simulink library "CommercialVehicleLibrary2G"  (R2021a)
settings: Solver=VariableStepAuto  StartTime=0.0  StopTime=10.0  RelTol=1e-3
values from neighbouring files (symbols this model uses):
  brake_input = [0   tmax ... (first row only)    [init_vehicle.m]    (also in run_Circle.m = [0  tmax; run_Coastdown.m = [0  2  tmax; run_DoubleLaneChangeDriver.m = [0   2  tmax; run_MaxAcc.m = [0  2  tmax)
  pose_t0 = [0 0 0 0]    [init_vehicle.m]    (also in run_Circle.m; run_Coastdown.m; run_DoubleLaneChangeDriver.m; run_MaxAcc.m)
  rdfname = 'TNO_FlatRoad.rdf'    [run_Circle.m]    (also in run_Coastdown.m; run_DoubleLaneChangeDriver.m; run_MaxAcc.m; run_Rollover.m)
  rdfname_inner = 'TNO_FlatRoad.rdf'    [run_Circle.m]    (also in run_Coastdown.m; run_DoubleLaneChangeDriver.m; run_MaxAcc.m; run_Rollover.m)
  steer_input = [0  tmax ... (first row only)    [init_vehicle.m]    (also in run_Circle.m = [0  2   10     13       tmax; run_Coastdown.m = [0 tmax; run_DoubleLaneChangeDriver.m = [0 tmax; run_MaxAcc.m = [0 tmax)
  throttle_input = [0         tmax ... (first row only)    [init_vehicle.m]    (also in run_Circle.m; run_Coastdown.m = [0        10         10.0001 tmax; run_DoubleLaneChangeDriver.m = [0        tmax; run_MaxAcc.m = [0        tmax)
  Vx = 0    [init_vehicle.m]    (also in run_Circle.m = Vx_kmh/3.6; run_Coastdown.m = Vx_kmh/3.6; run_DoubleLaneChangeDriver.m = Vx_kmh/3.6; run_MaxAcc.m)
  Vx_input = [0  tmax ... (first row only)    [init_vehicle.m]    (also in run_Circle.m; run_Coastdown.m = [0 tmax; run_DoubleLaneChangeDriver.m = [0 tmax; run_MaxAcc.m = [0 tmax)
undefined symbols (not defined in the file or in its folder): Drive, Floor, Fzstat, Fzstat1, Fzstat3, l, l_load1, l_load2, lbar, mass_load1, mass_load2, psi_semitrailer, rho, rim_Ixx, rim_Iyy, rim_mass, Steer, steer_path, tpfname, X, x_torsion, xcg, xcg1, xcg2, xcg_front, xcg_rear, xdrive1, xload1, xload2, xpos1, xref, xrev1, Xt0, Y, Yt0, Z
libraries: sm_lib x291, $bdroot x157, nesl_utility x143, vrlib x1
(part 10 of 12)

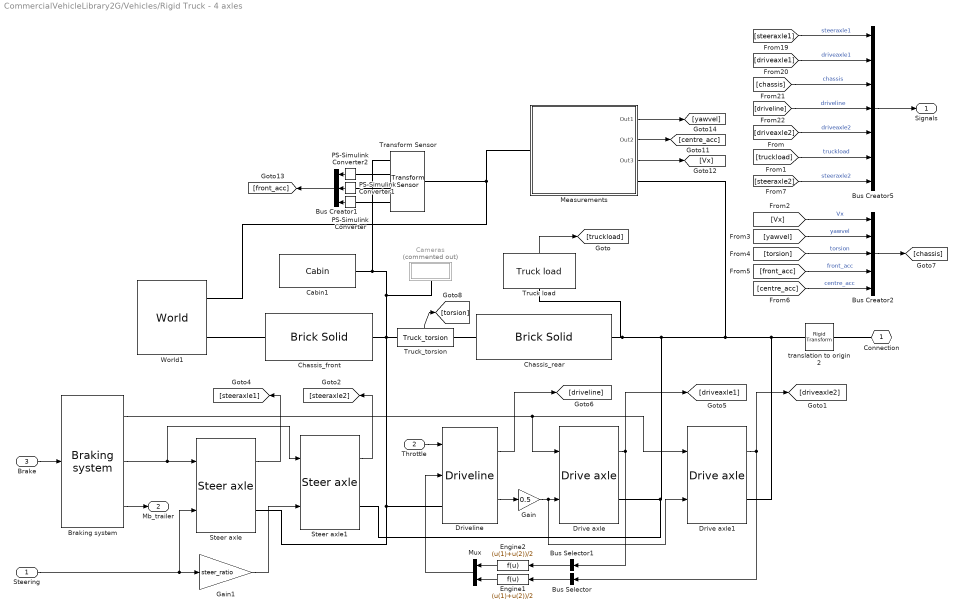
== system CommercialVehicleLibrary2G/Vehicles/Rigid Truck - 4 axles ==
  Steering : Inport
  Throttle : Inport  Port=2
  Brake : Inport  Port=3
  Braking system : $bdroot/Components/Braking system  SystemSampleTime=-1  VariantActivationTime=update diagram  Latency=0  AutoFrameSizeCalculation=off
  Bus Creator1 : BusCreator  Inputs=3
  Bus Creator2 : BusCreator  Inputs=5
  Bus Creator5 : BusCreator  Inputs=7
  Bus Selector : BusSelector  OutputSignals=Omega1,Omega2  OutputAsBus=on
  Bus Selector1 : BusSelector  OutputSignals=Omega1,Omega2  OutputAsBus=on
  Cabin1 : $bdroot/Assemblies/Cabin  xref=xref+1.10  zref=1.20
  Cameras : Subsystem  Commented=on
      settings: PortSchema="{\"entries\":[{\"content\":{\"sides\":[{\"content\":{\"connectorIds\":[]},\"type\":\"ConnectorPlacement.EquallySpacedRectSide\",\"uuid\":\"a276cb58-0a92-429b-8e88-be3307b37bb7\"},{\"content\":{\"connectorIds\":[],\"side\":\"RIGHT\"},\"type\":\"ConnectorPlacement.EquallySpacedRectSide\",\"uuid\":\"8a90bce0-2fe2-4c94-b803-8b8b0449a6a1\"},{\"content\":{\"connectorIds\":[],\"side\":\"TOP\"},\"type\":\"ConnectorPlacement.EquallySpacedRectSide\",\"uuid\":\"98d3107c-5bc7-4afe-b9f8-41acdc56c58c\"},{\"content\":{\"connectorIds\":[\"RConn1\"],\"side\":\"BOTTOM\"},\"type\":\"ConnectorPlacement.EquallySpacedRectSide\",\"uuid\":\"24ac9801-a810-4d3b-b9e2-6521fa5912b6\"}]},\"type\":\"ConnectorPlacement.EquallySpacedConnector\",\"uuid\":\"603d60ad-e553-44b7-87a5-94eb629e36a6\"}],\"packageUris\":[\"http://schema.mathworks.com/mf0/Connector/R2020b\"],\"version\":\"1.0\"}"
  Chassis_front : sm_lib/Body Elements/Brick Solid  GraphicAmbientColor=[0.15 0.15 0.15 1.0]  BasedOnType=Density  BrickDimensions=[l1 w1 h1]  BrickDimensionUnits=m  CenterOfMass=[0 0 0]  CenterOfMassUnits=m  GraphicDiffuseColor=[0.9 0.9 0.9]  Density=1000  DensityUnits=kg/m^3  DoExposeReferenceFrame=on  GraphicEmissiveColor=[0.0 0.0 0.0 1.0]  ExportEntireGeometry=off  SerializedFrames=<Frames><Frame><Id>Frame1</Id><Value><Name>F1</Name><Origin><Source>ReferenceFrame</Source><FeatureName></FeatureName></Origin><PrimaryAxis><DefinedDirection>+Z</DefinedDirection><Source>ReferenceFrame</Source><SourceDirection>+Z</SourceDirection><FeatureName></FeatureName></PrimaryAxis><SecondaryAxis><DefinedDirection>+X</DefinedDirection><Source>ReferenceFrame</Source><SourceDirection>+X</SourceDirection><FeatureName></FeatureName></SecondaryAxis></Value></Frame></Frames>  MarkerShape=Sphere  MarkerSize=10  GraphicType=FromGeometry  InertiaType=Custom  Mass=front_mass  MassUnits=kg  MomentsOfInertia=[front_Ixx front_Iyy front_Izz]  MomentsOfInertiaUnits=kg*m^2  GraphicOpacity=0.8  ProductsOfInertia=[0 0 0]  ProductsOfInertiaUnits=kg*m^2  GraphicShininess=75  GraphicSpecularColor=[0.5 0.5 0.5 1.0]  GraphicVisPropType=SimpleVisualProperties
  Chassis_rear : sm_lib/Body Elements/Brick Solid  GraphicAmbientColor=[0.15 0.15 0.15 1.0]  BasedOnType=Density  BrickDimensions=[l2 w2 h2]  BrickDimensionUnits=m  CenterOfMass=[0 0 0]  CenterOfMassUnits=m  GraphicDiffuseColor=[0.9 0.9 0.9]  Density=1000  DensityUnits=kg/m^3  DoExposeReferenceFrame=on  GraphicEmissiveColor=[0.0 0.0 0.0 1.0]  ExportEntireGeometry=off  SerializedFrames=<Frames><Frame><Id>Frame1</Id><Value><Name>F1</Name><Origin><Source>ReferenceFrame</Source><FeatureName></FeatureName></Origin><PrimaryAxis><DefinedDirection>+Z</DefinedDirection><Source>ReferenceFrame</Source><SourceDirection>+Z</SourceDirection><FeatureName></FeatureName></PrimaryAxis><SecondaryAxis><DefinedDirection>+X</DefinedDirection><Source>ReferenceFrame</Source><SourceDirection>+X</SourceDirection><FeatureName></FeatureName></SecondaryAxis></Value></Frame></Frames>  MarkerShape=Sphere  MarkerSize=10  GraphicType=FromGeometry  InertiaType=Custom  Mass=rear_mass  MassUnits=kg  MomentsOfInertia=[rear_Ixx rear_Iyy rear_Izz]  MomentsOfInertiaUnits=kg*m^2  GraphicOpacity=0.8  ProductsOfInertia=[0 0 0]  ProductsOfInertiaUnits=kg*m^2  GraphicShininess=75  GraphicSpecularColor=[0.5 0.5 0.5 1.0]  GraphicVisPropType=SimpleVisualProperties
  Drive axle : $bdroot/Assemblies/Drive axle  xpos=xdrive1  tpfname='truck1.tpf'  rdfname=rdfname  rdfname_inner=rdfname_inner  Vx=Vx  Fzstat=Fzstat3
  Drive axle1 : $bdroot/Assemblies/Drive axle  xpos=xdrive2  tpfname='truck1.tpf'  rdfname=rdfname  rdfname_inner=rdfname_inner  Vx=Vx  Fzstat=Fzstat4
  Driveline : $bdroot/Assemblies/Driveline  xref=xref-0.162  zref=0.58  param=DAF XEC + TC-Tronic (355 kW/2100 Nm)
  Engine1 : Fcn  Expr=(u(1)+u(2))/2
  Engine2 : Fcn  Expr=(u(1)+u(2))/2
  Gain : Gain  Gain=0.5
  Gain1 : Gain  Gain=steer_ratio
  Measurements : Subsystem
  Mux : Mux  Inputs=2
  PS-Simulink Converter : nesl_utility/PS-Simulink Converter  PhysicalDomain=network_engine_domain  SubClassName=ps_output  LeftPortType=input  RightPortType=output  PseudoPeriodic=off  Frequencies=[]  Unit=inherit  AffineConversion=off
  PS-Simulink Converter1 : nesl_utility/PS-Simulink Converter  PhysicalDomain=network_engine_domain  SubClassName=ps_output  LeftPortType=input  RightPortType=output  PseudoPeriodic=off  Frequencies=[]  Unit=inherit  AffineConversion=off
  PS-Simulink Converter2 : nesl_utility/PS-Simulink Converter  PhysicalDomain=network_engine_domain  SubClassName=ps_output  LeftPortType=input  RightPortType=output  PseudoPeriodic=off  Frequencies=[]  Unit=inherit  AffineConversion=off
  Steer axle : $bdroot/Assemblies/Steer axle  xpos=xref  tpfname='truck2b2.tpf'  rdfname=rdfname  Vx=Vx  Fzstat=Fzstat1
  Steer axle1 : $bdroot/Assemblies/Steer axle  xpos=xsteer2-xcg_rear  tpfname='truck2b2.tpf'  rdfname=rdfname  Vx=Vx  Fzstat=Fzstat2
  Transform Sensor : sm_lib/Frames and Transforms/Transform Sensor  MeasurementFrame=NonRotatingFollower  SenseAngle=off  SenseAxis=off  SenseAngle1=off  SenseAngle2=off  SenseAngle3=off  SenseQ=off  SenseR=off  SenseOmegaX=off  SenseOmegaY=off  SenseOmegaZ=off  SenseOmega1=off  SenseOmega2=off  SenseOmega3=off  SenseQDot=off  SenseRDot=off  SenseAlphaX=off  SenseAlphaY=off  SenseAlphaZ=off  SenseAlpha1=off  SenseAlpha2=off  SenseAlpha3=off  SenseQDDot=off  SenseRDDot=off  SenseX=off  SenseY=off  SenseZ=off  SenseRad=off  SenseAzim=off  SenseDist=off  SenseInc=off  SenseXDot=off  SenseYDot=off  SenseZDot=off  SenseRadDot=off  SenseAzimDot=off  SenseDistDot=off  SenseIncDot=off  SenseXDDot=on  SenseYDDot=on  SenseZDDot=on  SenseRadDDot=off  SenseAzimDDot=off  SenseDistDDot=off  SenseIncDDot=off
  Truck load : $bdroot/Assemblies/Truck load  xload=xload  zload=1.3  mass_load=mass_load  l_load=l_load  w=2.5  rho=rho
  Truck_torsion : $bdroot/Components/Truck_torsion  SystemSampleTime=-1  VariantActivationTime=update diagram  Latency=0  AutoFrameSizeCalculation=off
      settings: PortSchema="{\"entries\":[{\"content\":{\"sides\":[{\"content\":{\"connectorIds\":[\"LConn1\"]},\"type\":\"ConnectorPlacement.EquallySpacedRectSide\",\"uuid\":\"b43c74bd-af15-4ffb-863b-6a132848d787\"},{\"content\":{\"connectorIds\":[\"RConn1\"],\"side\":\"RIGHT\"},\"type\":\"ConnectorPlacement.EquallySpacedRectSide\",\"uuid\":\"8ef5ae9f-2f99-4b38-816f-c2fb0756fe1b\"},{\"content\":{\"connectorIds\":[\"Out1\"],\"side\":\"TOP\"},\"type\":\"ConnectorPlacement.EquallySpacedRectSide\",\"uuid\":\"649c363b-e78d-45fa-ac8c-bda3eda724e3\"}]},\"type\":\"ConnectorPlacement.EquallySpacedConnector\",\"uuid\":\"06fb9ebd-5177-4420-93bb-82569f181fb4\"}],\"packageUris\":[\"http://schema.mathworks.com/mf0/Connector/R2020b\"],\"version\":\"1.0\"}"
  World1 : $bdroot/Utilities/World  SystemSampleTime=-1  VariantActivationTime=update diagram  Latency=0  AutoFrameSizeCalculation=off
  translation to origin 2 : sm_lib/Frames and Transforms/Rigid Transform  TranslationMethod=Cartesian  TranslationStandardOffset=0  TranslationLengthUnit=m  TranslationStandardAxis=+Z  TranslationCartesianOffset=[-xcg_rear 0 -0.9]  TranslationROffset=0  TranslationROffsetUnits=m  TranslationZOffset=0  TranslationZOffsetUnits=m  TranslationThetaOffset=0  TranslationThetaOffsetUnits=deg  RotationMethod=None  RotationAngleUnits=deg  RotationStandardAxis=+Z  RotationAngle=0.0  RotationArbitraryAxis=[0 0 1]  FollAlignAxisA=+Z  BaseAlignAxisA=+X  FollAlignAxisB=+Y  BaseAlignAxisB=+Y  RotationSequenceAxes=FollowerAxes  RotationSequence=XYX  RotationSequenceAngles=[0 0 0]  RotationSequenceAnglesUnits=deg  RotationMatrix=[1 0 0; 0 1 0; 0 0 1]
  Connection : PMIOPort  Tag=PMCPort  Side=Right
  Signals : Outport
  Mb_trailer : Outport  Port=2
  wires:
  [yawvel] -> Bus Creator2/2  "yawvel"
  Bus Creator2/1 -> [chassis]
  [centre_acc] -> Bus Creator2/5  "centre_acc"
  [torsion] -> Bus Creator2/3  "torsion"
  [Vx] -> Bus Creator2/1  "Vx"
  [front_acc] -> Bus Creator2/4  "front_acc"
  Bus Creator1/1 -> [front_acc]
  PS-Simulink Converter2/1 -> Bus Creator1/1
  Truck_torsion/1 -> [torsion]
  PS-Simulink Converter/1 -> Bus Creator1/3
  Measurements/3(Out3) -> [Vx]
  Measurements/1(Out1) -> [yawvel]
  PS-Simulink Converter1/1 -> Bus Creator1/2
  Measurements/2(Out2) -> [centre_acc]
  Steer axle/1 -> [steeraxle1]
  Drive axle/1 -> [driveaxle1], Bus Selector1/1
  Braking system/3 -> Mb_trailer/1
  Brake/1 -> Braking system/1
  Throttle/1 -> Driveline/1
  Driveline/2 -> Gain/1
  Steering/1 -> Steer axle/2, Gain1/1
  Driveline/1 -> [driveline]
  [steeraxle1] -> Bus Creator5/1  "steeraxle1"
  [driveaxle1] -> Bus Creator5/2  "driveaxle1"
  [chassis] -> Bus Creator5/3  "chassis"
  [driveline] -> Bus Creator5/4  "driveline"
  Bus Creator5/1 -> Signals/1
  Braking system/1 -> Drive axle1/1, Drive axle/1
  Braking system/2 -> Steer axle1/1, Steer axle/1
  Drive axle1/1 -> [driveaxle2], Bus Selector/1
  [driveaxle2] -> Bus Creator5/5  "driveaxle2"
  Gain/1 -> Drive axle1/2, Drive axle/2
  Truck load/1 -> [truckload]
  [truckload] -> Bus Creator5/6  "truckload"
  Engine2/1 -> Mux/1
  Engine1/1 -> Mux/2
  Mux/1 -> Driveline/2
  Bus Selector1/1 -> Engine2/1
  Bus Selector/1 -> Engine1/1
  Gain1/1 -> Steer axle1/2
  Steer axle1/1 -> [steeraxle2]
  [steeraxle2] -> Bus Creator5/7  "steeraxle2"
  connections:
  Connection/RConn1 -- translation to origin 2/RConn1
  World1/RConn2 -- Chassis_front/RConn1
  Chassis_rear/RConn1 -- Truck_torsion/RConn1
  Transform Sensor/RConn2 -- PS-Simulink Converter2/LConn1
  PS-Simulink Converter/LConn1 -- Transform Sensor/RConn4
  PS-Simulink Converter1/LConn1 -- Transform Sensor/RConn3
  Measurements/LConn1 -- World1/RConn1 -- Transform Sensor/LConn1
  Cabin1/RConn1 -- Transform Sensor/RConn1 -- Cameras/RConn1 -- Steer axle/RConn1 -- Driveline/LConn1 -- Chassis_front/LConn1 -- Truck_torsion/LConn1
  Measurements/RConn1 -- Truck load/LConn1 -- Chassis_rear/LConn1 -- Steer axle1/RConn1 -- Drive axle/RConn1 -- Drive axle1/RConn1 -- translation to origin 2/LConn1

== system CommercialVehicleLibrary2G/Vehicles/Tractor ==
  Steering : Inport
  Throttle : Inport  Port=2
  Brake : Inport  Port=3
  Braking system : $bdroot/Components/Braking system  SystemSampleTime=-1  VariantActivationTime=update diagram  Latency=0  AutoFrameSizeCalculation=off
  Bus Creator1 : BusCreator  Inputs=3
  Bus Creator2 : BusCreator  Inputs=5
  Bus Creator5 : BusCreator  Inputs=4
  Bus Selector : BusSelector  OutputSignals=Omega1,Omega2  OutputAsBus=on
  Cabin : $bdroot/Assemblies/Cabin  xref=xref+1.10  zref=1.20
  Cameras : Subsystem  Commented=on
  Chassis_front : sm_lib/Body Elements/Brick Solid  GraphicAmbientColor=[0.15 0.15 0.15 1.0]  BasedOnType=Density  BrickDimensions=[l1 w1 h1]  BrickDimensionUnits=m  CenterOfMass=[0 0 0]  CenterOfMassUnits=m  GraphicDiffuseColor=[0.4 0.4 0.4]  Density=1000  DensityUnits=kg/m^3  DoExposeReferenceFrame=on  GraphicEmissiveColor=[0.0 0.0 0.0 1.0]  ExportEntireGeometry=off  SerializedFrames=<Frames><Frame><Id>Frame1</Id><Value><Name>F1</Name><Origin><Source>ReferenceFrame</Source><FeatureName></FeatureName></Origin><PrimaryAxis><DefinedDirection>+Z</DefinedDirection><Source>ReferenceFrame</Source><SourceDirection>+Z</SourceDirection><FeatureName></FeatureName></PrimaryAxis><SecondaryAxis><DefinedDirection>+X</DefinedDirection><Source>ReferenceFrame</Source><SourceDirection>+X</SourceDirection><FeatureName></FeatureName></SecondaryAxis></Value></Frame></Frames>  MarkerShape=Sphere  MarkerSize=10  GraphicType=FromGeometry  InertiaType=Custom  Mass=front_mass  MassUnits=kg  MomentsOfInertia=[front_Ixx front_Iyy front_Izz]  MomentsOfInertiaUnits=kg*m^2  GraphicOpacity=1  ProductsOfInertia=[0 0 0]  ProductsOfInertiaUnits=kg*m^2  GraphicShininess=75  GraphicSpecularColor=[0.5 0.5 0.5 1.0]  GraphicVisPropType=SimpleVisualProperties
  Chassis_rear : sm_lib/Body Elements/Brick Solid  GraphicAmbientColor=[0.15 0.15 0.15 1.0]  BasedOnType=Density  BrickDimensions=[l2 w2 h2]  BrickDimensionUnits=m  CenterOfMass=[0 0 0]  CenterOfMassUnits=m  GraphicDiffuseColor=[0.9 0.9 0.9]  Density=1000  DensityUnits=kg/m^3  DoExposeReferenceFrame=on  GraphicEmissiveColor=[0.0 0.0 0.0 1.0]  ExportEntireGeometry=off  SerializedFrames=<Frames><Frame><Id>Frame1</Id><Value><Name>F1</Name><Origin><Source>ReferenceFrame</Source><FeatureName></FeatureName></Origin><PrimaryAxis><DefinedDirection>+Z</DefinedDirection><Source>ReferenceFrame</Source><SourceDirection>+Z</SourceDirection><FeatureName></FeatureName></PrimaryAxis><SecondaryAxis><DefinedDirection>+X</DefinedDirection><Source>ReferenceFrame</Source><SourceDirection>+X</SourceDirection><FeatureName></FeatureName></SecondaryAxis></Value></Frame></Frames>  MarkerShape=Sphere  MarkerSize=10  GraphicType=FromGeometry  InertiaType=Custom  Mass=rear_mass  MassUnits=kg  MomentsOfInertia=[rear_Ixx rear_Iyy rear_Izz]  MomentsOfInertiaUnits=kg*m^2  GraphicOpacity=0.8  ProductsOfInertia=[0 0 0]  ProductsOfInertiaUnits=kg*m^2  GraphicShininess=75  GraphicSpecularColor=[0.5 0.5 0.5 1.0]  GraphicVisPropType=SimpleVisualProperties
  Drive axle : $bdroot/Assemblies/Drive axle  xpos=xref+xrear  tpfname='truck1.tpf'  rdfname=rdfname  rdfname_inner=rdfname_inner  Vx=Vx  Fzstat=Fzstat2
  Driveline : $bdroot/Assemblies/Driveline  xref=xref-0.162  zref=0.58  param=DAF XEC + TC-Tronic (355 kW/2100 Nm)
  Measurements : Subsystem
  PS-Simulink Converter : nesl_utility/PS-Simulink Converter  PhysicalDomain=network_engine_domain  SubClassName=ps_output  LeftPortType=input  RightPortType=output  PseudoPeriodic=off  Frequencies=[]  Unit=inherit  AffineConversion=off
  PS-Simulink Converter1 : nesl_utility/PS-Simulink Converter  PhysicalDomain=network_engine_domain  SubClassName=ps_output  LeftPortType=input  RightPortType=output  PseudoPeriodic=off  Frequencies=[]  Unit=inherit  AffineConversion=off
  PS-Simulink Converter2 : nesl_utility/PS-Simulink Converter  PhysicalDomain=network_engine_domain  SubClassName=ps_output  LeftPortType=input  RightPortType=output  PseudoPeriodic=off  Frequencies=[]  Unit=inherit  AffineConversion=off
  Steer axle : $bdroot/Assemblies/Steer axle  xpos=xref  tpfname='truck2b2.tpf'  rdfname=rdfname  Vx=Vx  Fzstat=Fzstat1
  Tractor_torsion : $bdroot/Components/Tractor_torsion  SystemSampleTime=-1  VariantActivationTime=update diagram  Latency=0  AutoFrameSizeCalculation=off
      settings: PortSchema="{\"entries\":[{\"content\":{\"sides\":[{\"content\":{\"connectorIds\":[\"LConn1\"]},\"type\":\"ConnectorPlacement.EquallySpacedRectSide\",\"uuid\":\"b43c74bd-af15-4ffb-863b-6a132848d787\"},{\"content\":{\"connectorIds\":[\"RConn1\"],\"side\":\"RIGHT\"},\"type\":\"ConnectorPlacement.EquallySpacedRectSide\",\"uuid\":\"8ef5ae9f-2f99-4b38-816f-c2fb0756fe1b\"},{\"content\":{\"connectorIds\":[\"Out1\"],\"side\":\"TOP\"},\"type\":\"ConnectorPlacement.EquallySpacedRectSide\",\"uuid\":\"649c363b-e78d-45fa-ac8c-bda3eda724e3\"}]},\"type\":\"ConnectorPlacement.EquallySpacedConnector\",\"uuid\":\"06fb9ebd-5177-4420-93bb-82569f181fb4\"}],\"packageUris\":[\"http://schema.mathworks.com/mf0/Connector/R2020b\"],\"version\":\"1.0\"}"
  Transform Sensor : sm_lib/Frames and Transforms/Transform Sensor  MeasurementFrame=NonRotatingFollower  SenseAngle=off  SenseAxis=off  SenseAngle1=off  SenseAngle2=off  SenseAngle3=off  SenseQ=off  SenseR=off  SenseOmegaX=off  SenseOmegaY=off  SenseOmegaZ=off  SenseOmega1=off  SenseOmega2=off  SenseOmega3=off  SenseQDot=off  SenseRDot=off  SenseAlphaX=off  SenseAlphaY=off  SenseAlphaZ=off  SenseAlpha1=off  SenseAlpha2=off  SenseAlpha3=off  SenseQDDot=off  SenseRDDot=off  SenseX=off  SenseY=off  SenseZ=off  SenseRad=off  SenseAzim=off  SenseDist=off  SenseInc=off  SenseXDot=off  SenseYDot=off  SenseZDot=off  SenseRadDot=off  SenseAzimDot=off  SenseDistDot=off  SenseIncDot=off  SenseXDDot=on  SenseYDDot=on  SenseZDDot=on  SenseRadDDot=off  SenseAzimDDot=off  SenseDistDDot=off  SenseIncDDot=off
  World : $bdroot/Utilities/World  SystemSampleTime=-1  VariantActivationTime=update diagram  Latency=0  AutoFrameSizeCalculation=off
  translation to origin : sm_lib/Frames and Transforms/Rigid Transform  TranslationMethod=Cartesian  TranslationStandardOffset=0  TranslationLengthUnit=m  TranslationStandardAxis=+Z  TranslationCartesianOffset=[-xcg_rear 0 -0.9]  TranslationROffset=0  TranslationROffsetUnits=m  TranslationZOffset=0  TranslationZOffsetUnits=m  TranslationThetaOffset=0  TranslationThetaOffsetUnits=deg  RotationMethod=None  RotationAngleUnits=deg  RotationStandardAxis=+Z  RotationAngle=0.0  RotationArbitraryAxis=[0 0 1]  FollAlignAxisA=+Z  BaseAlignAxisA=+X  FollAlignAxisB=+Y  BaseAlignAxisB=+Y  RotationSequenceAxes=FollowerAxes  RotationSequence=XYX  RotationSequenceAngles=[0 0 0]  RotationSequenceAnglesUnits=deg  RotationMatrix=[1 0 0; 0 1 0; 0 0 1]
  5th Wheel : PMIOPort  Tag=PMCPort  Side=Right
  Signals : Outport
  Mb_trailer : Outport  Port=2
  wires:
  Braking system/2 -> Steer axle/1
  Braking system/1 -> Drive axle/1
  Bus Creator5/1 -> Signals/1
  [driveline] -> Bus Creator5/4  "driveline"
  [chassis] -> Bus Creator5/3  "chassis"
  [driveaxle] -> Bus Creator5/2  "driveaxle"
  [steeraxle] -> Bus Creator5/1  "steeraxle"
  Driveline/1 -> [driveline]
  Steering/1 -> Steer axle/2
  Driveline/2 -> Drive axle/2
  Bus Selector/1 -> Driveline/2
  Throttle/1 -> Driveline/1
  Brake/1 -> Braking system/1
  Braking system/3 -> Mb_trailer/1
  Drive axle/1 -> Bus Selector/1, [driveaxle]
  Steer axle/1 -> [steeraxle]
  Measurements/2(Out2) -> [centre_acc]
  PS-Simulink Converter1/1 -> Bus Creator1/2
  Measurements/1(Out1) -> [yawvel]
  Measurements/3(Out3) -> [Vx]
  PS-Simulink Converter/1 -> Bus Creator1/3
  Tractor_torsion/1 -> [torsion]
  PS-Simulink Converter2/1 -> Bus Creator1/1
  Bus Creator1/1 -> [front_acc]
  [front_acc] -> Bus Creator2/4  "front_acc"
  [Vx] -> Bus Creator2/1  "Vx"
  [torsion] -> Bus Creator2/3  "torsion"
  [centre_acc] -> Bus Creator2/5  "centre_acc"
  Bus Creator2/1 -> [chassis]
  [yawvel] -> Bus Creator2/2  "yawvel"
  connections:
  Cabin/RConn1 -- Cameras/LConn1 -- Transform Sensor/RConn1 -- Chassis_front/LConn1 -- Tractor_torsion/LConn1 -- Driveline/LConn1 -- Steer axle/RConn1
  Transform Sensor/LConn1 -- World/RConn1 -- Measurements/LConn1
  translation to origin/LConn1 -- Drive axle/RConn1 -- Chassis_rear/LConn1 -- Measurements/RConn1
  PS-Simulink Converter1/LConn1 -- Transform Sensor/RConn3
  PS-Simulink Converter/LConn1 -- Transform Sensor/RConn4
  Transform Sensor/RConn2 -- PS-Simulink Converter2/LConn1
  Chassis_rear/RConn1 -- Tractor_torsion/RConn1
  World/RConn2 -- Chassis_front/RConn1
  5th Wheel/RConn1 -- translation to origin/RConn1

== system CommercialVehicleLibrary2G/Assemblies/Cabin/Subsystem ==
  External Force and Torque : sm_lib/Forces and Torques/External Force and Torque  ForceResolutionFrame=AttachedFrame  EnableForceX=on  EnableForceY=off  EnableForceZ=off  EnableForce=off  TorqueResolutionFrame=AttachedFrame  EnableTorqueX=off  EnableTorqueY=off  EnableTorqueZ=off  EnableTorque=off
  Fcn : Fcn  Expr=-0.5*1.23*0.6*10.5*u(1)*abs(u(1))
  File Solid : sm_lib/Body Elements/File Solid  ExtGeomFileName=E:\Thesis\Original TST Model\Cabin.stl  UnitType=Custom  ExtGeomFileUnits=mm  StepReaderType=HEX  ExportConvexHullGeometry=off  InertiaType=Custom  Mass=1e-09  MassUnits=kg  CenterOfMass=[0 0 0]  CenterOfMassUnits=m  MomentsOfInertia=[1 1 1]  MomentsOfInertiaUnits=kg*m^2  ProductsOfInertia=[0 0 0]  ProductsOfInertiaUnits=kg*m^2  BasedOnType=DensityFromFile  Density=1000  DensityUnits=kg/m^3  DoExposeReferenceFrame=on  SerializedFrames=<Frames/>  GraphicType=FromGeometry  MarkerShape=Sphere  MarkerSize=10  GraphicVisPropType=SimpleVisualProperties  GraphicDiffuseColor=[0.4 0.4 0.4]  GraphicSpecularColor=[0.5 0.5 0.5 1.0]  GraphicAmbientColor=[0.15 0.15 0.15 1.0]  GraphicEmissiveColor=[0.0 0.0 0.0 1.0]  GraphicShininess=75  GraphicOpacity=1.0
  PS-Simulink Converter : nesl_utility/PS-Simulink Converter  PhysicalDomain=network_engine_domain  SubClassName=ps_output  LeftPortType=input  RightPortType=output  PseudoPeriodic=off  Frequencies=[]  Unit=inherit  AffineConversion=off
  Rigid Transform : sm_lib/Frames and Transforms/Rigid Transform  TranslationMethod=None  TranslationStandardOffset=0  TranslationLengthUnit=m  TranslationStandardAxis=+Z  TranslationCartesianOffset=[0 0 0]  TranslationROffset=0  TranslationROffsetUnits=m  TranslationZOffset=0  TranslationZOffsetUnits=m  TranslationThetaOffset=0  TranslationThetaOffsetUnits=deg  RotationMethod=StandardAxis  RotationAngleUnits=deg  RotationStandardAxis=+X  RotationAngle=90  RotationArbitraryAxis=[0 0 1]  FollAlignAxisA=+X  BaseAlignAxisA=+Y  FollAlignAxisB=+Y  BaseAlignAxisB=+Z  RotationSequenceAxes=FollowerAxes  RotationSequence=XYX  RotationSequenceAngles=[0 0 0]  RotationSequenceAnglesUnits=deg  RotationMatrix=[1 0 0; 0 1 0; 0 0 1]
  Rigid Transform3 : sm_lib/Frames and Transforms/Rigid Transform  TranslationMethod=None  TranslationStandardOffset=0  TranslationLengthUnit=m  TranslationStandardAxis=+Z  TranslationCartesianOffset=[0 0 0]  TranslationROffset=0  TranslationROffsetUnits=m  TranslationZOffset=0  TranslationZOffsetUnits=m  TranslationThetaOffset=0  TranslationThetaOffsetUnits=deg  RotationMethod=StandardAxis  RotationAngleUnits=deg  RotationStandardAxis=+Y  RotationAngle=90  RotationArbitraryAxis=[0 0 1]  FollAlignAxisA=+X  BaseAlignAxisA=+Y  FollAlignAxisB=+Y  BaseAlignAxisB=+Z  RotationSequenceAxes=FollowerAxes  RotationSequence=XYX  RotationSequenceAngles=[0 0 0]  RotationSequenceAnglesUnits=deg  RotationMatrix=[1 0 0; 0 1 0; 0 0 1]
  Rigid Transform4 : sm_lib/Frames and Transforms/Rigid Transform  TranslationMethod=Cartesian  TranslationStandardOffset=0  TranslationLengthUnit=m  TranslationStandardAxis=+Z  TranslationCartesianOffset=[0.15 -2.55 -1.75]  TranslationROffset=0  TranslationROffsetUnits=m  TranslationZOffset=0  TranslationZOffsetUnits=m  TranslationThetaOffset=0  TranslationThetaOffsetUnits=deg  RotationMethod=None  RotationAngleUnits=deg  RotationStandardAxis=+Y  RotationAngle=90  RotationArbitraryAxis=[0 0 1]  FollAlignAxisA=+X  BaseAlignAxisA=+Y  FollAlignAxisB=+Y  BaseAlignAxisB=+Z  RotationSequenceAxes=FollowerAxes  RotationSequence=XYX  RotationSequenceAngles=[0 0 0]  RotationSequenceAnglesUnits=deg  RotationMatrix=[1 0 0; 0 1 0; 0 0 1]
  Simulink-PS Converter : nesl_utility/Simulink-PS Converter  PhysicalDomain=network_engine_domain  SubClassName=ps_input  LeftPortType=input  RightPortType=output  PseudoPeriodic=off  Frequencies=[]  NoiseDistribution=none  NoiseParameters=[]  Unit=1  AffineConversion=off  FilteringAndDerivatives=provide  SimscapeFilterOrder=1  InputFilterTimeConstant=0.001  UdotUserProvided=0
  Transform Sensor : sm_lib/Frames and Transforms/Transform Sensor  MeasurementFrame=NonRotatingFollower  SenseAngle=off  SenseAxis=off  SenseAngle1=off  SenseAngle2=off  SenseAngle3=off  SenseQ=off  SenseR=off  SenseOmegaX=off  SenseOmegaY=off  SenseOmegaZ=off  SenseOmega1=off  SenseOmega2=off  SenseOmega3=off  SenseQDot=off  SenseRDot=off  SenseAlphaX=off  SenseAlphaY=off  SenseAlphaZ=off  SenseAlpha1=off  SenseAlpha2=off  SenseAlpha3=off  SenseQDDot=off  SenseRDDot=off  SenseX=off  SenseY=off  SenseZ=off  SenseRad=off  SenseAzim=off  SenseDist=off  SenseInc=off  SenseXDot=on  SenseYDot=off  SenseZDot=off  SenseRadDot=off  SenseAzimDot=off  SenseDistDot=off  SenseIncDot=off  SenseXDDot=off  SenseYDDot=off  SenseZDDot=off  SenseRadDDot=off  SenseAzimDDot=off  SenseDistDDot=off  SenseIncDDot=off
  World Frame : sm_lib/Frames and Transforms/World Frame
  Conn1 : PMIOPort  Side=Left
  wires:
  PS-Simulink Converter/1 -> Fcn/1
  Fcn/1 -> Simulink-PS Converter/1
  connections:
  Rigid Transform3/RConn1 -- Rigid Transform4/LConn1
  External Force and Torque/RConn1 -- File Solid/RConn1 -- Rigid Transform4/RConn1
  Transform Sensor/LConn1 -- World Frame/RConn1
  Simulink-PS Converter/RConn1 -- External Force and Torque/LConn1
  Transform Sensor/RConn1 -- Rigid Transform/LConn1 -- Conn1/RConn1
  PS-Simulink Converter/LConn1 -- Transform Sensor/RConn2
  Rigid Transform/RConn1 -- Rigid Transform3/LConn1

== system CommercialVehicleLibrary2G/Assemblies/Drive axle/Wheel 1 L ==
  MF Tyre L : $bdroot/Components/MF Tyre L  Tag=SimMechanics Wheel + tyre  idtyre=1  inertia=[rim_mass rim_Ixx rim_Iyy]  tpfname=tpfname  rdfname=rdfname  side_mode=(1xxx) left  cnt_mode=(x1xx) smooth road  dyn_mode=(xx1x) relaxation behaviour  mf_mode=(xxx4) combined  use_mode=1e8  disp_debug=off
  Non-moving road : $bdroot/Utilities/Non-moving road  Tag=Non-moving road  dummy=off
  Scaling factors : $bdroot/Utilities/Scaling factors  Tag=Scaling factors  LMUX=1  LKX=1  LMUY=1  LKY=1  LKYC=1  LTR=1  LKZC=1
  "Terminator " : Terminator
  B : PMIOPort  Side=Left
  Out1 : Outport
  wires:
  Non-moving road/1 -> MF Tyre L/1
  Scaling factors/1 -> MF Tyre L/2
  MF Tyre L/1 -> Out1/1
  MF Tyre L/2 -> "Terminator "/1
  connections:
  MF Tyre L/LConn1 -- B/RConn1

== system CommercialVehicleLibrary2G/Assemblies/Drive axle/Wheel 2 L ==
  2nd Wheel offset : sm_lib/Frames and Transforms/Rigid Transform  TranslationMethod=StandardAxis  TranslationStandardOffset=-ywhl  TranslationLengthUnit=m  TranslationStandardAxis=+Z  TranslationCartesianOffset=[0 0 0]  TranslationROffset=0  TranslationROffsetUnits=m  TranslationZOffset=0  TranslationZOffsetUnits=m  TranslationThetaOffset=0  TranslationThetaOffsetUnits=deg  RotationMethod=None  RotationAngleUnits=deg  RotationStandardAxis=+Z  RotationAngle=0.0  RotationArbitraryAxis=[0 0 1]  FollAlignAxisA=+X  BaseAlignAxisA=+Y  FollAlignAxisB=+Y  BaseAlignAxisB=+Z  RotationSequenceAxes=FollowerAxes  RotationSequence=XYX  RotationSequenceAngles=[0 0 0]  RotationSequenceAnglesUnits=deg  RotationMatrix=[1 0 0; 0 1 0; 0 0 1]
  MF Tyre L : $bdroot/Components/MF Tyre L  Tag=SimMechanics Wheel + tyre  idtyre=1  inertia=[rim_mass rim_Ixx rim_Iyy]  tpfname=tpfname  rdfname=rdfname  side_mode=(1xxx) left  cnt_mode=(x1xx) smooth road  dyn_mode=(xx1x) relaxation behaviour  mf_mode=(xxx4) combined  use_mode=1e8  disp_debug=off
  Non-moving road : $bdroot/Utilities/Non-moving road  Tag=Non-moving road  dummy=off
  Scaling factors : $bdroot/Utilities/Scaling factors  Tag=Scaling factors  LMUX=1  LKX=1  LMUY=1  LKY=1  LKYC=1  LTR=1  LKZC=1
  "Terminator " : Terminator
  B : PMIOPort  Side=Left
  Out1 : Outport
  wires:
  MF Tyre L/2 -> "Terminator "/1
  MF Tyre L/1 -> Out1/1
  Scaling factors/1 -> MF Tyre L/2
  Non-moving road/1 -> MF Tyre L/1
  connections:
  MF Tyre L/LConn1 -- 2nd Wheel offset/RConn1
  2nd Wheel offset/LConn1 -- B/RConn1

== system CommercialVehicleLibrary2G/Assemblies/Drive axle/Wheel1 R ==
  MF Tyre R : $bdroot/Components/MF Tyre R  Tag=SimMechanics Wheel + tyre  idtyre=2  inertia=[rim_mass rim_Ixx rim_Iyy]  tpfname=tpfname  rdfname=rdfname  side_mode=(2xxx) right  cnt_mode=(x1xx) smooth road  dyn_mode=(xx1x) relaxation behaviour  mf_mode=(xxx4) combined  use_mode=1e8  disp_debug=off
  Non-moving road : $bdroot/Utilities/Non-moving road  Tag=Non-moving road  dummy=off
  Scaling factors : $bdroot/Utilities/Scaling factors  Tag=Scaling factors  LMUX=1  LKX=1  LMUY=1  LKY=1  LKYC=1  LTR=1  LKZC=1
  Terminator 3 : Terminator
  B : PMIOPort  Side=Left
  Out1 : Outport
  wires:
  MF Tyre R/2 -> Terminator 3/1
  MF Tyre R/1 -> Out1/1
  Non-moving road/1 -> MF Tyre R/1
  Scaling factors/1 -> MF Tyre R/2
  connections:
  B/RConn1 -- MF Tyre R/LConn1

== system CommercialVehicleLibrary2G/Assemblies/Drive axle/Wheel2 R ==
  2nd Wheel offset : sm_lib/Frames and Transforms/Rigid Transform  TranslationMethod=StandardAxis  TranslationStandardOffset=ywhl  TranslationLengthUnit=m  TranslationStandardAxis=+Z  TranslationCartesianOffset=[0 0 0]  TranslationROffset=0  TranslationROffsetUnits=m  TranslationZOffset=0  TranslationZOffsetUnits=m  TranslationThetaOffset=0  TranslationThetaOffsetUnits=deg  RotationMethod=None  RotationAngleUnits=deg  RotationStandardAxis=+Z  RotationAngle=0.0  RotationArbitraryAxis=[0 0 1]  FollAlignAxisA=+X  BaseAlignAxisA=+Y  FollAlignAxisB=+Y  BaseAlignAxisB=+Z  RotationSequenceAxes=FollowerAxes  RotationSequence=XYX  RotationSequenceAngles=[0 0 0]  RotationSequenceAnglesUnits=deg  RotationMatrix=[1 0 0; 0 1 0; 0 0 1]
  MF Tyre R : $bdroot/Components/MF Tyre R  Tag=SimMechanics Wheel + tyre  idtyre=2  inertia=[rim_mass rim_Ixx rim_Iyy]  tpfname=tpfname  rdfname=rdfname  side_mode=(2xxx) right  cnt_mode=(x1xx) smooth road  dyn_mode=(xx1x) relaxation behaviour  mf_mode=(xxx4) combined  use_mode=1e8  disp_debug=off
  Non-moving road : $bdroot/Utilities/Non-moving road  Tag=Non-moving road  dummy=off
  Scaling factors : $bdroot/Utilities/Scaling factors  Tag=Scaling factors  LMUX=1  LKX=1  LMUY=1  LKY=1  LKYC=1  LTR=1  LKZC=1
  "Terminator " : Terminator
  B : PMIOPort  Side=Left
  Out1 : Outport
  wires:
  MF Tyre R/1 -> Out1/1
  MF Tyre R/2 -> "Terminator "/1
  Non-moving road/1 -> MF Tyre R/1
  Scaling factors/1 -> MF Tyre R/2
  connections:
  2nd Wheel offset/LConn1 -- B/RConn1
  2nd Wheel offset/RConn1 -- MF Tyre R/LConn1

== system CommercialVehicleLibrary2G/Assemblies/Driveline/engine and differential ==
  throttle : Inport
  omega_wheels : Inport  Port=2
  Bus Creator : BusCreator  Inputs=2
  Demux : Demux  Outputs=2
  Engine : Fcn  Expr=eng_power/(abs(u)+1e-10)
  Mux : Mux  Inputs=2
  Product2 : Product  Inputs=3  InputSameDT=on  SaturateOnIntegerOverflow=on  OutDataTypeStr=Inherit: Same as first input
  Saturation : Saturate  UpperLimit=max_engine_torque*first_gear_ratio  LowerLimit=0
  Saturation1 : Saturate  UpperLimit=1  LowerLimit=-0.2
  Scope : Scope
  Sum : Sum  Inputs=|++
  differential1 : Gain  Gain=0.5*final_drive_ratio
  differential2 : Gain  Gain=0.5*final_drive_ratio
  rev. limiter : Lookup  InputValues="[-0.2*omega_max  0.9*omega_max omega_max 2*omega_max]"  Table=[1 1 0 0]
  Md_wheels : Outport
  signals : Outport  Port=2
  wires:
  [omega] -> Bus Creator/2  "omega"
  [throttle] -> Bus Creator/1  "throttle"
  Bus Creator/1 -> signals/1
  Demux/2 -> Sum/2
  Demux/1 -> Sum/1
  omega_wheels/1 -> Demux/1
  Engine/1 -> Saturation/1
  throttle/1 -> Scope/1, Saturation1/1
  Mux/1 -> Md_wheels/1
  differential2/1 -> Mux/1, Mux/2
  Saturation1/1 -> [throttle], Product2/1
  Saturation/1 -> Product2/2
  Sum/1 -> differential1/1
  differential1/1 -> [omega], rev. limiter/1, Engine/1
  Product2/1 -> differential2/1
  rev. limiter/1 -> Product2/3

== system CommercialVehicleLibrary2G/Assemblies/Driver/CruiseControl ==
  Vx,ref : Inport
  Vx,actual : Inport  Port=2
  Add : Sum  Inputs=+-
  Add1 : Sum
  Gain : Gain  Gain=5
  Gain1 : Gain  Gain=5
  Integrator : Integrator  InitialCondition=0.0  LimitOutput=on  UpperSaturationLimit=0.1  LowerSaturationLimit=-0.1
  Lookup Table : Lookup  InputValues="[-10  2  10 30]"  Table=[0.04 0.04 1 1]
  Product : Product  RndMeth=Zero
  Product1 : Product  RndMeth=Zero
  Transfer Fcn : TransferFcn  Denominator=[0.16 1]
  throttle : Outport  VectorParamsAs1DForOutWhenUnconnected=off
  wires:
  Vx,actual/1 -> Add/2, Transfer Fcn/1
  Vx,ref/1 -> Add/1
  Gain1/1 -> Integrator/1
  Integrator/1 -> Add1/2
  Gain/1 -> Add1/1
  Add1/1 -> throttle/1
  Add/1 -> Product/1, Product1/1
  Product/1 -> Gain/1
  Product1/1 -> Gain1/1
  Lookup Table/1 -> Product1/2, Product/2
  Transfer Fcn/1 -> Lookup Table/1

== system CommercialVehicleLibrary2G/Assemblies/Driver/PreviewSteering ==
  FrontAxlePos : Inport
  RearAxlePos : Inport  Port=2
  Vx : Inport  Port=3
  Constant : Constant  Value=10
  Constant1 : Constant  Value=driver_path'
  Embedded MATLAB Function : MATLAB Function  TreatAsAtomicUnit=on
  Fcn : Fcn  Expr=atan2( u(1), u(2) )
  Gain : Gain  Gain=-steer_ratio*steer_sens
  Gain1 : Gain  Gain=[1 1 0]
  Gain2 : Gain  Gain=lookahead_time
  Memory1 : Memory  InitialCondition=-1
  Mux : Mux  Inputs=2
  Normalize Vector : vrlib/Utilities/Normalize Vector  maxzero=0
  Product : Product  RndMeth=Zero
  Saturation : Saturate  UpperLimit=100  LowerLimit=5
  Sum : Sum  Inputs=|++
  Sum1 : Sum  Inputs=+-|
  To Workspace2 : ToWorkspace  VariableName=p_driver_pos  SampleTime=-1
  To Workspace3 : ToWorkspace  VariableName=p_driver_viewpoint  SampleTime=-1
  To Workspace4 : ToWorkspace  VariableName=p_dist  SampleTime=-1
  To Workspace5 : ToWorkspace  VariableName=p_frontaxle_pos  SampleTime=-1
  Transfer Fcn : TransferFcn  Denominator=[0.01 1]
  steer angle (rad) : Outport
  wires:
  Transfer Fcn/1 -> steer angle (rad)/1
  Mux/1 -> Fcn/1
  Saturation/1 -> Mux/2, Product/2
  Vx/1 -> Gain2/1
  FrontAxlePos/1 -> Sum1/1, To Workspace5/1, Sum/1
  RearAxlePos/1 -> Sum1/2
  Gain1/1 -> To Workspace3/1, Embedded MATLAB Function/2(point)
  Embedded MATLAB Function/2(pos) -> To Workspace2/1
  Constant1/1 -> Embedded MATLAB Function/1(line)
  Embedded MATLAB Function/1(dist) -> Mux/1, To Workspace4/1
  Sum/1 -> Gain1/1
  Constant/1 -> Embedded MATLAB Function/3(npoints)
  Memory1/1 -> Embedded MATLAB Function/4(idx1)
  Embedded MATLAB Function/3(idx2) -> Memory1/1
  Gain/1 -> Transfer Fcn/1
  Fcn/1 -> Gain/1
  Gain2/1 -> Saturation/1
  Product/1 -> Sum/2
  Normalize Vector/1 -> Product/1
  Sum1/1 -> Normalize Vector/1

== system CommercialVehicleLibrary2G/Combinations/LZV_B/To_workspace_semitrailer1 ==
  note: Axle 1
  note: Axle 2
  note: Axle 3
  note: Tyres & Omega
  In1 : Inport
  Bus Selector1 : BusSelector  OutputSignals=axle1.Axle_roll  OutputAsBus=on
  Bus Selector11 : BusSelector  OutputSignals=axle3.Axle_acc  OutputAsBus=on
  Bus Selector2 : BusSelector  OutputSignals=axle2.Axle_pos  OutputAsBus=on
  Bus Selector22 : BusSelector  OutputSignals=axle3.Axle_pos  OutputAsBus=on
  Bus Selector3 : BusSelector  OutputSignals=axle2.Axle_acc  OutputAsBus=on
  Bus Selector4 : BusSelector  OutputSignals=axle2.Axle_roll  OutputAsBus=on
  Bus Selector5 : BusSelector  OutputSignals=axle1.Axle_pos  OutputAsBus=on
  Bus Selector6 : BusSelector  OutputSignals=axle1.Axle_acc  OutputAsBus=on
  Bus Selector7 : BusSelector  OutputSignals=axle3.Axle_roll  OutputAsBus=on
  Subsystem : Subsystem
  Subsystem1 : Subsystem
  Subsystem2 : Subsystem
  Subsystem3 : Subsystem
  To Workspace1 : ToWorkspace  VariableName=p_semitraileraxle3_pos  SampleTime=-1
  To Workspace10 : ToWorkspace  VariableName=p_semitraileraxle2_pos  SampleTime=-1
  To Workspace11 : ToWorkspace  VariableName=p_semitraileraxle2_acc  SampleTime=-1
  To Workspace2 : ToWorkspace  VariableName=p_semitraileraxle3_acc  SampleTime=-1
  To Workspace3 : ToWorkspace  VariableName=p_semitraileraxle3_roll  SampleTime=-1
  To Workspace30 : ToWorkspace  VariableName=p_semitrailer_Fx  SampleTime=-1
  To Workspace31 : ToWorkspace  VariableName=p_semitrailer_Fy  SampleTime=-1
  To Workspace4 : ToWorkspace  VariableName=p_semitraileraxle1_roll  SampleTime=-1
  To Workspace5 : ToWorkspace  VariableName=p_semitraileraxle1_pos  SampleTime=-1
  To Workspace6 : ToWorkspace  VariableName=p_semitraileraxle1_acc  SampleTime=-1
  To Workspace7 : ToWorkspace  VariableName=p_semitrailer_omega  SampleTime=-1
  To Workspace8 : ToWorkspace  VariableName=p_semitraileraxle2_roll  SampleTime=-1
  To Workspace9 : ToWorkspace  VariableName=p_semitrailer_Fz  SampleTime=-1
  wires:
  Bus Selector22/1 -> To Workspace1/1
  Bus Selector6/1 -> To Workspace6/1
  Bus Selector5/1 -> To Workspace5/1
  Subsystem3/1(Out1) -> To Workspace7/1
  Subsystem2/1(Out1) -> To Workspace9/1
  Subsystem1/1(Out1) -> To Workspace31/1
  Subsystem/1(Out1) -> To Workspace30/1
  Bus Selector3/1 -> To Workspace11/1
  Bus Selector2/1 -> To Workspace10/1
  Bus Selector11/1 -> To Workspace2/1
  Bus Selector1/1 -> To Workspace4/1
  Bus Selector4/1 -> To Workspace8/1
  In1/1 -> Bus Selector3/1, Bus Selector2/1, Bus Selector5/1, Bus Selector7/1, Subsystem3/1(In1), Subsystem2/1(In1), Subsystem1/1(In1), Bus Selector22/1, Subsystem/1(In1), Bus Selector11/1, Bus Selector4/1, Bus Selector1/1, Bus Selector6/1
  Bus Selector7/1 -> To Workspace3/1

== system CommercialVehicleLibrary2G/Combinations/LZV_B/To_workspace_semitrailer2 ==
  note: Tyres & Omega
  note: Axle 3
  note: Axle 2
  note: Axle 1
  In1 : Inport
  Bus Selector1 : BusSelector  OutputSignals=axle1.Axle_roll  OutputAsBus=on
  Bus Selector11 : BusSelector  OutputSignals=axle3.Axle_acc  OutputAsBus=on
  Bus Selector2 : BusSelector  OutputSignals=axle2.Axle_pos  OutputAsBus=on
  Bus Selector22 : BusSelector  OutputSignals=axle3.Axle_pos  OutputAsBus=on
  Bus Selector3 : BusSelector  OutputSignals=axle2.Axle_acc  OutputAsBus=on
  Bus Selector4 : BusSelector  OutputSignals=axle2.Axle_roll  OutputAsBus=on
  Bus Selector5 : BusSelector  OutputSignals=axle1.Axle_pos  OutputAsBus=on
  Bus Selector6 : BusSelector  OutputSignals=axle1.Axle_acc  OutputAsBus=on
  Bus Selector7 : BusSelector  OutputSignals=axle3.Axle_roll  OutputAsBus=on
  Subsystem : Subsystem
  Subsystem1 : Subsystem
  Subsystem2 : Subsystem
  Subsystem3 : Subsystem
  To Workspace1 : ToWorkspace  VariableName=p_semitrailer2axle3_pos  SampleTime=-1
  To Workspace10 : ToWorkspace  VariableName=p_semitrailer2axle2_pos  SampleTime=-1
  To Workspace11 : ToWorkspace  VariableName=p_semitrailer2axle2_acc  SampleTime=-1
  To Workspace2 : ToWorkspace  VariableName=p_semitrailer2axle3_acc  SampleTime=-1
  To Workspace3 : ToWorkspace  VariableName=p_semitrailer2axle3_roll  SampleTime=-1
  To Workspace30 : ToWorkspace  VariableName=p_semitrailer2_Fx  SampleTime=-1
  To Workspace31 : ToWorkspace  VariableName=p_semitrailer2_Fy  SampleTime=-1
  To Workspace4 : ToWorkspace  VariableName=p_semitrailer2axle1_roll  SampleTime=-1
  To Workspace5 : ToWorkspace  VariableName=p_semitrailer2axle1_pos  SampleTime=-1
  To Workspace6 : ToWorkspace  VariableName=p_semitrailer2axle1_acc  SampleTime=-1
  To Workspace7 : ToWorkspace  VariableName=p_semitrailer2_omega  SampleTime=-1
  To Workspace8 : ToWorkspace  VariableName=p_semitrailer2axle2_roll  SampleTime=-1
  To Workspace9 : ToWorkspace  VariableName=p_semitrailer2_Fz  SampleTime=-1
  wires:
  Bus Selector7/1 -> To Workspace3/1
  In1/1 -> Bus Selector6/1, Bus Selector1/1, Bus Selector4/1, Bus Selector11/1, Subsystem/1(In1), Bus Selector22/1, Subsystem1/1(In1), Subsystem2/1(In1), Subsystem3/1(In1), Bus Selector7/1, Bus Selector5/1, Bus Selector2/1, Bus Selector3/1
  Bus Selector4/1 -> To Workspace8/1
  Bus Selector1/1 -> To Workspace4/1
  Bus Selector11/1 -> To Workspace2/1
  Bus Selector2/1 -> To Workspace10/1
  Bus Selector3/1 -> To Workspace11/1
  Subsystem/1(Out1) -> To Workspace30/1
  Subsystem1/1(Out1) -> To Workspace31/1
  Subsystem2/1(Out1) -> To Workspace9/1
  Subsystem3/1(Out1) -> To Workspace7/1
  Bus Selector5/1 -> To Workspace5/1
  Bus Selector6/1 -> To Workspace6/1
  Bus Selector22/1 -> To Workspace1/1

== system CommercialVehicleLibrary2G/Combinations/LZV_E/To_workspace_drawbar_trailer_2axle 2 ==
  note: Axle 1
  note: Axle 2
  note: Chassis & Load
  note: Tyres & Omega
  In1 : Inport
  Bus Selector10 : BusSelector  OutputSignals=axle1.Axle_roll  OutputAsBus=on
  Bus Selector11 : BusSelector  OutputSignals=trailerload.acc_center  OutputAsBus=on
  Bus Selector12 : BusSelector  OutputSignals=axle2.Axle_acc  OutputAsBus=on
  Bus Selector2 : BusSelector  OutputSignals=axle2.Axle_pos  OutputAsBus=on
  Bus Selector22 : BusSelector  OutputSignals=trailerload.pos  OutputAsBus=on
  Bus Selector3 : BusSelector  OutputSignals=axle2.Axle_roll  OutputAsBus=on
  Bus Selector5 : BusSelector  OutputSignals=axle1.Axle_pos  OutputAsBus=on
  Bus Selector6 : BusSelector  OutputSignals=axle1.Axle_acc  OutputAsBus=on
  Bus Selector7 : BusSelector  OutputSignals=trailerload.acc_corner  OutputAsBus=on
  Subsystem : Subsystem
  Subsystem1 : Subsystem
  Subsystem2 : Subsystem
  Subsystem3 : Subsystem
  To Workspace1 : ToWorkspace  VariableName=p_trailer2_load_pos  SampleTime=-1
  To Workspace10 : ToWorkspace  VariableName=p_trailer2_axle2_acc  SampleTime=-1
  To Workspace2 : ToWorkspace  VariableName=p_trailer2_load_acc_center  SampleTime=-1
  To Workspace23 : ToWorkspace  VariableName=p_trailer2_axle1_roll  SampleTime=-1
  To Workspace3 : ToWorkspace  VariableName=p_trailer2_load_acc_corner  SampleTime=-1
  To Workspace30 : ToWorkspace  VariableName=p_trailer2_Fx  SampleTime=-1
  To Workspace31 : ToWorkspace  VariableName=p_trailer2_Fy  SampleTime=-1
  To Workspace4 : ToWorkspace  VariableName=p_trailer2_axle2_roll  SampleTime=-1
  To Workspace5 : ToWorkspace  VariableName=p_trailer2_axle1_pos  SampleTime=-1
  To Workspace6 : ToWorkspace  VariableName=p_trailer2_axle1_acc  SampleTime=-1
  To Workspace7 : ToWorkspace  VariableName=p_trailer2_omega  SampleTime=-1
  To Workspace8 : ToWorkspace  VariableName=p_trailer2_axle2_pos  SampleTime=-1
  To Workspace9 : ToWorkspace  VariableName=p_trailer2_Fz  SampleTime=-1
  wires:
  Bus Selector7/1 -> To Workspace3/1
  Bus Selector10/1 -> To Workspace23/1
  Bus Selector22/1 -> To Workspace1/1
  In1/1 -> Bus Selector3/1, Bus Selector2/1, Bus Selector5/1, Bus Selector12/1, Bus Selector10/1, Subsystem3/1(In1), Bus Selector7/1, Subsystem2/1(In1), Subsystem1/1(In1), Bus Selector22/1, Subsystem/1(In1), Bus Selector11/1, Bus Selector6/1
  Bus Selector12/1 -> To Workspace10/1
  Bus Selector6/1 -> To Workspace6/1
  Bus Selector5/1 -> To Workspace5/1
  Subsystem3/1(Out1) -> To Workspace7/1
  Subsystem2/1(Out1) -> To Workspace9/1
  Subsystem1/1(Out1) -> To Workspace31/1
  Subsystem/1(Out1) -> To Workspace30/1
  Bus Selector3/1 -> To Workspace4/1
  Bus Selector2/1 -> To Workspace8/1
  Bus Selector11/1 -> To Workspace2/1

== system CommercialVehicleLibrary2G/Components/Brake//Wheel_bearing/Rotational joint around y axis ==
  Torque : Inport
  PS-Simulink Converter : nesl_utility/PS-Simulink Converter  PhysicalDomain=network_engine_domain  SubClassName=ps_output  LeftPortType=input  RightPortType=output  PseudoPeriodic=off  Frequencies=[]  Unit=inherit  AffineConversion=off
  Revolute Joint : sm_lib/Joints/Revolute Joint  JointMode=Normal  SenseConstraintForce=off  SenseConstraintForceX=off  SenseConstraintForceY=off  SenseConstraintForceZ=off  SenseConstraintTorque=off  SenseConstraintTorqueX=off  SenseConstraintTorqueY=off  SenseConstraintTorqueZ=off  SenseTotalForce=off  SenseTotalForceX=off  SenseTotalForceY=off  SenseTotalForceZ=off  SenseTotalTorque=off  SenseTotalTorqueX=off  SenseTotalTorqueY=off  SenseTotalTorqueZ=off  CompositeWrenchDir=FollowerOnBase  CompositeWrenchFrame=BaseFrame  EquilibriumPosition=0  EquilibriumPositionUnits=deg  SpringStiffness=0  SpringStiffnessUnits=N*m/deg  DampingCoefficient=0  DampingCoefficientUnits=N*m/(deg/s)  TorqueActuationMode=InputTorque  MotionActuationMode=ComputedMotion  SensePosition=off  SenseVelocity=on  SenseAcceleration=off  SenseTorqueForce=off  SenseLowerLimitTorqueForce=off  SenseUpperLimitTorqueForce=off  LowerLimitSpecify=off  LowerLimitBound=-90  LowerLimitBoundUnits=deg  LowerLimitStiffness=1e4  LowerLimitStiffnessUnits=N*m/deg  LowerLimitDamping=10  LowerLimitDampingUnits=N*m/(deg/s)  LowerLimitTransitionRegionWidth=0.1  LowerLimitTransitionRegionWidthUnits=deg  UpperLimitSpecify=off  UpperLimitBound=90  UpperLimitBoundUnits=deg  UpperLimitStiffness=1e4  UpperLimitStiffnessUnits=N*m/deg  UpperLimitDamping=10  UpperLimitDampingUnits=N*m/(deg/s)  UpperLimitTransitionRegionWidth=0.1  UpperLimitTransitionRegionWidthUnits=deg  PositionTargetSpecify=off  PositionTargetPriority=High  PositionTargetValue=0  PositionTargetValueUnits=deg  VelocityTargetSpecify=on  VelocityTargetPriority=High  VelocityTargetValue=Vx/radius  VelocityTargetValueUnits=rad/s
  Rigid Transform : sm_lib/Frames and Transforms/Rigid Transform  TranslationMethod=None  TranslationStandardOffset=0  TranslationLengthUnit=m  TranslationStandardAxis=+Z  TranslationCartesianOffset=[0 0 0]  TranslationROffset=0  TranslationROffsetUnits=m  TranslationZOffset=0  TranslationZOffsetUnits=m  TranslationThetaOffset=0  TranslationThetaOffsetUnits=deg  RotationMethod=AlignedAxes  RotationAngleUnits=deg  RotationStandardAxis=+Z  RotationAngle=0.0  RotationArbitraryAxis=[0 0 1]  FollAlignAxisA=+Z  BaseAlignAxisA=+Y  FollAlignAxisB=+X  BaseAlignAxisB=+X  RotationSequenceAxes=FollowerAxes  RotationSequence=XYX  RotationSequenceAngles=[0 0 0]  RotationSequenceAnglesUnits=deg  RotationMatrix=[1 0 0; 0 1 0; 0 0 1]
  Rigid Transform1 : sm_lib/Frames and Transforms/Rigid Transform  TranslationMethod=None  TranslationStandardOffset=0  TranslationLengthUnit=m  TranslationStandardAxis=+Z  TranslationCartesianOffset=[0 0 0]  TranslationROffset=0  TranslationROffsetUnits=m  TranslationZOffset=0  TranslationZOffsetUnits=m  TranslationThetaOffset=0  TranslationThetaOffsetUnits=deg  RotationMethod=None  RotationAngleUnits=deg  RotationStandardAxis=+Z  RotationAngle=0.0  RotationArbitraryAxis=[0 0 1]  FollAlignAxisA=+Y  BaseAlignAxisA=+Z  FollAlignAxisB=+X  BaseAlignAxisB=+X  RotationSequenceAxes=FollowerAxes  RotationSequence=XYX  RotationSequenceAngles=[0 0 0]  RotationSequenceAnglesUnits=deg  RotationMatrix=[1 0 0; 0 1 0; 0 0 1]
  Simulink-PS Converter : nesl_utility/Simulink-PS Converter  PhysicalDomain=network_engine_domain  SubClassName=ps_input  LeftPortType=input  RightPortType=output  PseudoPeriodic=off  Frequencies=[]  NoiseDistribution=none  NoiseParameters=[]  Unit=1  AffineConversion=off  FilteringAndDerivatives=filter  SimscapeFilterOrder=2  InputFilterTimeConstant=0.001  UdotUserProvided=0
  Axle : PMIOPort  Side=Left
  Wheel : PMIOPort  Port=2  Side=Right
  Rotational speed : Outport
  wires:
  PS-Simulink Converter/1 -> Rotational speed/1
  Torque/1 -> Simulink-PS Converter/1
  connections:
  Wheel/RConn1 -- Rigid Transform1/RConn1
  Rigid Transform1/LConn1 -- Revolute Joint/RConn1
  PS-Simulink Converter/LConn1 -- Revolute Joint/RConn2
  Simulink-PS Converter/RConn1 -- Revolute Joint/LConn2
  Rigid Transform/LConn1 -- Axle/RConn1
  Revolute Joint/LConn1 -- Rigid Transform/RConn1
